simulink model "sun"  (R2020a)
settings: Solver=FixedStepAuto  StartTime=0.0  StopTime=19  FixedStep=0.01  RelTol=1e-3
model workspace (MAT data in the model file):
  a = 6
  cb = 0.9
  d = 268
  lat = 23.5
  local_meridian = 80
  long = 130
  nmmpt = 0.98
  npanel = 0.25
  sc = 1
  solar_noon = 12.4333333333
libraries: simulink_extras x2, simulink x1
settings Model: OrderedModelArguments=off  Creator=user  LastModifiedBy=user

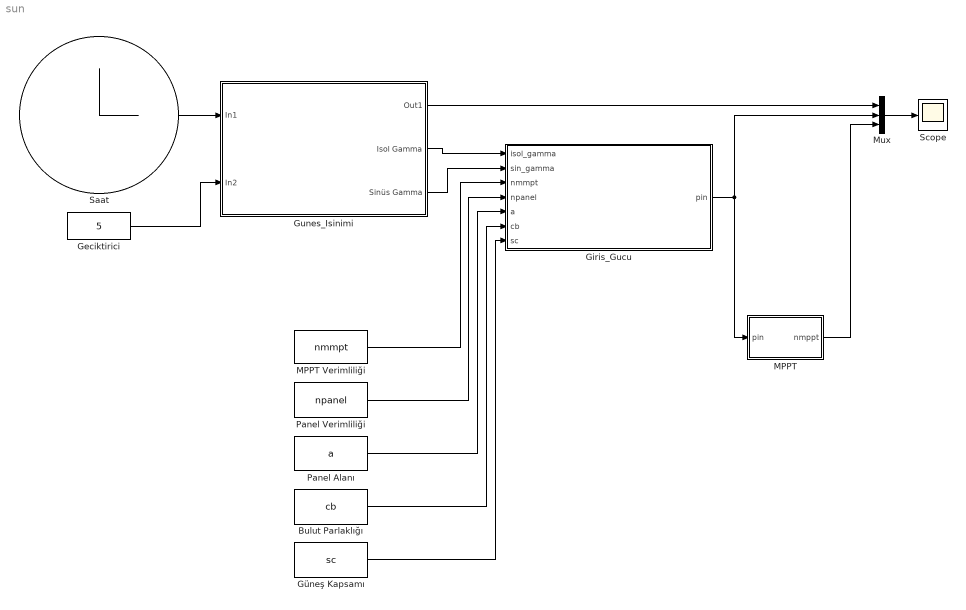
== system sun ==
  Bulut Parlaklığı : Constant  Value=cb
  Geciktirici : Constant  Value=5
  Giris_Gucu : MATLAB Function  TreatAsAtomicUnit=on
  Gunes_Isinimi : Subsystem
      mask Display: image("C:\Users\user\Desktop\gunes.jpg")
  Güneş Kapsamı : Constant  Value=sc
  MPPT : MATLAB Function  TreatAsAtomicUnit=on
  MPPT Verimliliği : Constant  Value=nmmpt
  Mux : Mux  Inputs=3
  Panel Alanı : Constant  Value=a
  Panel Verimliliği : Constant  Value=npanel
  Saat : Clock
      settings: Decimation=5
  Scope : Scope
  wires:
  Saat/1 -> Gunes_Isinimi/1(In1)
  Geciktirici/1 -> Gunes_Isinimi/2(In2)
  Gunes_Isinimi/2(Isol Gamma) -> Giris_Gucu/1(isol_gamma)
  Gunes_Isinimi/3(Sinüs Gamma) -> Giris_Gucu/2(sin_gamma)
  Panel Verimliliği/1 -> Giris_Gucu/4(npanel)
  Panel Alanı/1 -> Giris_Gucu/5(a)
  Bulut Parlaklığı/1 -> Giris_Gucu/6(cb)
  Güneş Kapsamı/1 -> Giris_Gucu/7(sc)
  Gunes_Isinimi/1(Out1) -> Mux/1
  Giris_Gucu/1(pin) -> MPPT/1(pin), Mux/2
  Mux/1 -> Scope/1
  MPPT Verimliliği/1 -> Giris_Gucu/3(nmmpt)
  MPPT/1(nmppt) -> Mux/3

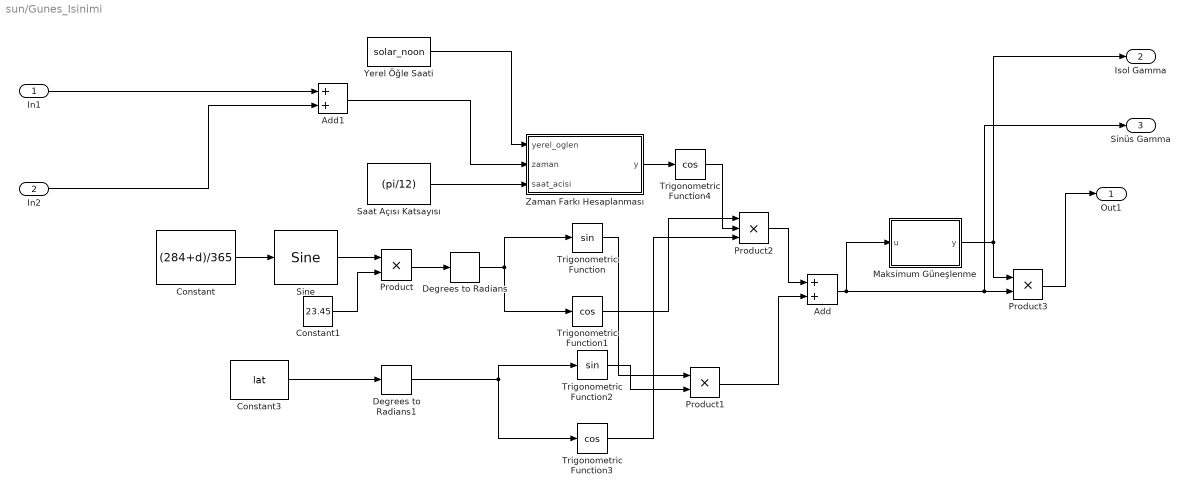
== system sun/Gunes_Isinimi ==
  In1 : Inport
  In2 : Inport  Port=2
  Add : Sum
  Add1 : Sum
  Constant : Constant  Value=(284+d)/365
  Constant1 : Constant  Value=23.45
  Constant3 : Constant  Value=lat
  Degrees to Radians : simulink_extras/Transformations/Degrees to Radians
  Degrees to Radians1 : simulink_extras/Transformations/Degrees to Radians
  Maksimum Güneşlenme : MATLAB Function  TreatAsAtomicUnit=on
  Product : Product
  Product1 : Product
  Product2 : Product  Inputs=3
  Product3 : Product
  Saat Açısı Katsayısı : Constant  Value=(pi/12)
  Sine : simulink/Lookup Tables/Sine  Formula=sin(2*pi*u)  NumDataPoints=(2^5)+1  OutputWordLength=16  InternalRulePriority=Speed
  Trigonometric Function : Trigonometry
  Trigonometric Function1 : Trigonometry  Operator=cos
  Trigonometric Function2 : Trigonometry
  Trigonometric Function3 : Trigonometry  Operator=cos
  Trigonometric Function4 : Trigonometry  Operator=cos
  Yerel Öğle Saati : Constant  Value=solar_noon
  Zaman Farkı Hesaplanması : MATLAB Function  TreatAsAtomicUnit=on
  Out1 : Outport
  Isol Gamma : Outport  Port=2
  Sinüs Gamma : Outport  Port=3
  wires:
  Degrees to Radians1/1 -> Trigonometric Function3/1, Trigonometric Function2/1
  Add1/1 -> Zaman Farkı Hesaplanması/2(zaman)
  Saat Açısı Katsayısı/1 -> Zaman Farkı Hesaplanması/3(saat_acisi)
  In1/1 -> Add1/1
  Constant1/1 -> Product/2
  Sine/1 -> Product/1
  Maksimum Güneşlenme/1(y) -> Isol Gamma/1, Product3/1
  Zaman Farkı Hesaplanması/1(y) -> Trigonometric Function4/1
  Trigonometric Function4/1 -> Product2/2
  Constant/1 -> Sine/1
  Add/1 -> Maksimum Güneşlenme/1(u), Sinüs Gamma/1, Product3/2
  Degrees to Radians/1 -> Trigonometric Function1/1, Trigonometric Function/1
  Product/1 -> Degrees to Radians/1
  Trigonometric Function3/1 -> Product2/3
  Product1/1 -> Add/2
  Trigonometric Function2/1 -> Product1/2
  Product2/1 -> Add/1
  Trigonometric Function1/1 -> Product2/1
  Yerel Öğle Saati/1 -> Zaman Farkı Hesaplanması/1(yerel_oglen)
  Constant3/1 -> Degrees to Radians1/1
  Trigonometric Function/1 -> Product1/1
  In2/1 -> Add1/2
  Product3/1 -> Out1/1

== matlab function sun/Giris_Gucu ==
  data: isol_gamma input; pin output; sin_gamma input; nmmpt input; npanel input; a input; cb input; sc input
function pin = fcn(isol_gamma,sin_gamma, nmmpt  , npanel, a, cb, sc)
pin=npanel*nmmpt*a*(sc*sin_gamma+(1-sc)*cb)*isol_gamma;

== matlab function sun/Gunes_Isinimi/Zaman Farkı Hesaplanması ==
  data: yerel_oglen input; zaman input; y output; saat_acisi input
function y = fcn(yerel_oglen, zaman, saat_acisi)
c1=(zaman - (yerel_oglen));
y = c1*saat_acisi;

== matlab function sun/MPPT ==
  data: pin input; nmppt output
function nmppt = fcn(pin)
nmppt = 100*atan(0.225*pin)-0.003*pin+0.8;

== matlab function sun/Gunes_Isinimi/Maksimum Güneşlenme ==
  data: u input; y output
function y = fcn(u)
m=1 ./ u;
k=1353* 0.687 ^ (power(complex(m),0.678));
if imag(k)==0
    y=real(k);
else
    y=0;
end
